simulink model "crossroad_cs_old"  (R2021a)
settings: Solver=ode5  StartTime=0.0  StopTime=50  FixedStep=1/1000  RelTol=1e-3
PreLoadFcn:
  | mbxruntime.callbacks.PreLoadFcn(bdroot);
PostLoadFcn:
  | mbxruntime.callbacks.PostLoadFcn(bdroot);
InitFcn:
  | mbxruntime.callbacks.InitFcn(bdroot);
StartFcn:
  | mbxruntime.callbacks.StartFcn(bdroot);
StopFcn:
  | mbxruntime.callbacks.StopFcn(bdroot);
model workspace: external: MAT-File .\crossroad_cs_hws.mat (data not in the file)
values from neighbouring files (symbols this model uses):
  c_factor = 43.75    [emplanner_init.m]
  cf = -175016    [emplanner_init.m]
  cr = -130634    [emplanner_init.m]
  KD_PID_distance = 0.0    (= 0)    [emplanner_init.m]
  KD_PID_speed = 0    [emplanner_init.m]
  KI_PID_distance = 0.0    (= 0)    [emplanner_init.m]
  KI_PID_speed = 0    [emplanner_init.m]
  KP_PID_distance = 0.5    [emplanner_init.m]
  KP_PID_speed = 1.8    [emplanner_init.m]
  la = 1.265    [emplanner_init.m]
  lb = 2.947-1.265    (= 1.682)    [emplanner_init.m]
  LQR_K1 = k(:,1)'    [emplanner_init.m]
  LQR_K2 = k(:,2)'    [emplanner_init.m]
  LQR_K3 = k(:,3)'    [emplanner_init.m]
  LQR_K4 = k(:,4)'    [emplanner_init.m]
  m = 2020    [emplanner_init.m]
  my_global_path_x = [0.4409 0.940746626271 1.44028225507 1.93950267328 2.43840536558 2.93698884522 3.43525224935 3.93319509352 4.43081712279 4.92811822143 5.42509835808 5.92175755256 ... (6001 elements, 6001x1)]    [my_global_path.mat]    (also in my_global_path_200.mat = [0.4409 0.940746626271 1.44028225507 1.93950267328 2.4384053)
  my_global_path_y = [58.2244 58.2243999975 58.2243999675 58.2243998683 58.224399668 58.2243993499 58.2243989099 58.2243983526 58.2243976886 58.2243969324 58.2243961011 58.2243952132 ... (6001 elements, 6001x1)]    [my_global_path.mat]    (also in my_global_path_200.mat = [58.2244 58.2243999975 58.2243999675 58.2243998683 58.224399)
  rack_displacement = [-39.14 , -37.2 , -35.29 , -33.43 , -31.6 , -29.81 , -28.06 , -26.34 , -24.66 ,      -23.01 , -21.38 , -19.79 , -18.23 , -16.69 , -15.18 , -13.7 , -12.23 , -10.8 , -9.38 , -7.98 ,     -6.61 , -5.25 , -3.91 , -2.59 , -1.29 , 0 , 1.27 , 2.54 , 3.78 , 5.02 , 6.24 , 7.46 , 8.66 ,      9.86 , 11.05 , 12.24 , 13.41 , 14.59 , 15.76 , 16.92 , 18.09 , 19.25 , 20.42 , 21.59 , 22.76 ,      23.93 , 25.11 , 26 ...(+26 chars)    [emplanner_init.m]
  right_wheel_ground = [-70 ,-67.2 , -64.4 , -61.6 , -58.8 , -56 , -53.2 , -50.4 , -47.6 , -44.8 , -42 ,      -39.2 , -36.4 , -33.6 , -30.8 , -28 , -25.2 , -22.4 , -19.6 , -16.8 , -14 , -11.2 , -8.4 , -5.6 ,      -2.8 , 0 , 2.8 , 5.6 , 8.4 , 11.2 , 14 , 16.8 , 19.6 , 22.4 , 25.2 , 28 , 30.8 , 33.6 , 36.4 ,      39.2 , 42 , 44.8 , 47.6 , 50.4 , 53.2 , 56 , 58.8 , 61.6 , 64.4 , 67.2 , 70 ]    [emplanner_init.m]
  vx_break_point = zeros(1,5000)    [emplanner_init.m]
undefined symbols (not defined in the file or in its folder): aubr, DiscIntNeverNeededParam, tablebr, vubr
libraries: PreScanSimulinkLibrary x11, Solver_SF x1
(part 3 of 8)

== system crossroad_cs_old/Audi_A8_Sedan_1/Dynamics_UserSpecified/MuxState ==
  note: mode: Dynamics
  note: mode: Positioning
  note: mode: Dynamics
      | VelVEHICLE
      | wrt VEH
  note: AnglesVEHICLE
      | wrtGLOB
  note: For state mode 'Dynamic' positions
      | are not taken into account, as they
      | are computed by integrating velocity.
      | Click annotation for Help.
  x [m] : Inport  SampleTime=TimeStep
  y [m] : Inport  Port=2  SampleTime=TimeStep
  z [m] : Inport  Port=3  SampleTime=TimeStep
  dx [m/s] : Inport  Port=4  SampleTime=TimeStep
  dy [m/s] : Inport  Port=5  SampleTime=TimeStep
  dz [m/s] : Inport  Port=6  SampleTime=TimeStep
  R [rad] : Inport  Port=7  SampleTime=TimeStep
  P [rad] : Inport  Port=8  SampleTime=TimeStep
  Y [rad] : Inport  Port=9  SampleTime=TimeStep
  Constant : Constant  DisableCoverage=on  Value=positioningmode
  Discrete-Time Integrator : DiscreteIntegrator  SampleTime=TimeStep  ICPrevOutput=DiscIntNeverNeededParam  ICPrevScaledInput=DiscIntNeverNeededParam
  Ground : Ground
  Ground1 : Ground
  Mux1 : Mux  Inputs=[3 3]
  Mux2 : Mux  Inputs=3
  Mux3 : Mux  Inputs=3
  Mux4 : Mux  Inputs=3
  Mux5 : Mux  Inputs=[3 3]
  Mux6 : Mux  Inputs=[6 3]
  Switch : Switch  Threshold=0.5
  Transformation_BODY2GLOBAL : PreScanSimulinkLibrary/Simple_Vehicle_Dynamics/Chassis/MuxDynState/Transformation_BODY2GLOBAL  SystemSampleTime=-1  VariantActivationTime=update diagram  Latency=0  AutoFrameSizeCalculation=off
  mux3 : Mux  Inputs=3
  state : Outport
  wires:
  Constant/1 -> Switch/2
  Mux6/1 -> state/1
  Mux4/1 -> Mux1/1
  Mux5/1 -> Switch/3
  Mux1/1 -> Switch/1
  Switch/1 -> Mux6/1  "PosVeh wrt  GLOB"
  P [rad]/1 -> Mux3/2
  R [rad]/1 -> Mux3/1
  dz [m/s]/1 -> Mux2/3
  dy [m/s]/1 -> Mux2/2
  dx [m/s]/1 -> Mux2/1
  z [m]/1 -> Mux4/3
  y [m]/1 -> Mux4/2
  x [m]/1 -> Mux4/1
  Ground1/1 -> mux3/2  "pitch"
  Y [rad]/1 -> mux3/3, Mux3/3  "yaw"
  Mux3/1 -> Mux6/2
  Transformation_BODY2GLOBAL/1 -> Discrete-Time Integrator/1, Mux5/2  "VelVEH wrt  GLOB"
  mux3/1 -> Transformation_BODY2GLOBAL/2
  Ground/1 -> mux3/1  "roll"
  Mux2/1 -> Mux1/2, Transformation_BODY2GLOBAL/1
  Discrete-Time Integrator/1 -> Mux5/1  "PosVEH wrt  GLOB"

== system crossroad_cs_old/Audi_A8_Sedan_1/Dynamics_UserSpecified/STATE_Audi_A8_Sedan_1 ==
  State : Inport  SampleTime=TimeStep
  Bus Creator : BusCreator  Inputs=15  OutDataTypeStr=Bus: PRESCAN_STATEACTUATORDATA  NonVirtualBus=on
  Constant : Constant  Value=0
  Demux : Demux  Outputs=15
  Mux : Mux  Inputs=3
  Mux1 : Mux  Inputs=3
  Mux2 : Mux  Inputs=3
  iniBODYAngles wrtVEH [rad] : Constant  Value=Roll0  SampleTime=TimeStep
  iniBODYAngles wrtVEH [rad]1 : Constant  Value=Pitch0  SampleTime=TimeStep
  iniVEHAngles wrtGLOB [rad] : Constant  Value=Yaw0  SampleTime=TimeStep
  iniVEHposition wrtGLOB [m] : Constant  Value=x0  SampleTime=TimeStep
  iniVEHposition wrtGLOB [m]1 : Constant  Value=y0  SampleTime=TimeStep
  iniVEHposition wrtGLOB [m]2 : Constant  Value=z0  SampleTime=TimeStep
  state2FullState : PreScanSimulinkLibrary/state2FullState  SystemSampleTime=-1  VariantActivationTime=update diagram  Latency=0  AutoFrameSizeCalculation=off
  StateBus : Outport  OutDataTypeStr=Bus: PRESCAN_STATEACTUATORDATA
  wires:
  Mux2/1 -> state2FullState/4
  iniVEHAngles wrtGLOB [rad]/1 -> Mux2/3
  Mux1/1 -> state2FullState/3
  Constant/1 -> Mux2/1, Mux2/2, Mux1/3
  iniBODYAngles wrtVEH [rad]1/1 -> Mux1/2
  iniBODYAngles wrtVEH [rad]/1 -> Mux1/1
  Mux/1 -> state2FullState/2
  iniVEHposition wrtGLOB [m]2/1 -> Mux/3
  iniVEHposition wrtGLOB [m]/1 -> Mux/1
  iniVEHposition wrtGLOB [m]1/1 -> Mux/2
  Demux/15 -> Bus Creator/15  "AngularVelocityYaw"
  Demux/14 -> Bus Creator/14  "AngularVelocityPitch"
  Demux/13 -> Bus Creator/13  "AngularVelocityRoll"
  Demux/12 -> Bus Creator/12  "OrientationYaw"
  Demux/11 -> Bus Creator/11  "OrientationPitch"
  Demux/10 -> Bus Creator/10  "OrientationRoll"
  Demux/9 -> Bus Creator/9  "AccelerationZ"
  Demux/8 -> Bus Creator/8  "AccelerationY"
  Demux/7 -> Bus Creator/7  "AccelerationX"
  Demux/6 -> Bus Creator/6  "VelocityZ"
  Demux/5 -> Bus Creator/5  "VelocityY"
  Demux/4 -> Bus Creator/4  "VelocityX"
  Demux/3 -> Bus Creator/3  "PositionZ"
  Demux/2 -> Bus Creator/2  "PositionY"
  Demux/1 -> Bus Creator/1  "PositionX"
  state2FullState/1 -> Demux/1
  State/1 -> state2FullState/1
  Bus Creator/1 -> StateBus/1

== system crossroad_cs_old/Audi_A8_Sedan_1/SELF_Demux/compas converter ==
  rotz [rad] : Inport
  cart2compas : Subsystem
  rad2deg : Gain  Gain=180/pi
  heading [deg] : Outport
  wires:
  rad2deg/1 -> cart2compas/1(Angle [deg])
  rotz [rad]/1 -> rad2deg/1
  cart2compas/1(heading [deg]) -> heading [deg]/1

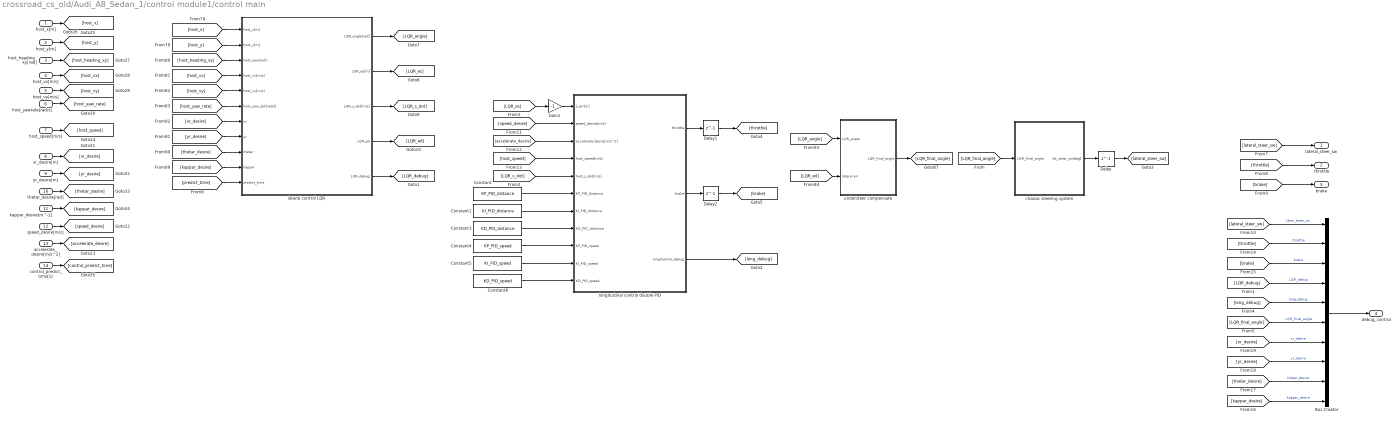
== system crossroad_cs_old/Audi_A8_Sedan_1/control module1/control main ==
  host_x[m] : Inport
  host_y[m] : Inport  Port=2
  host_heading_xy[rad] : Inport  Port=3
  host_vx[m/s] : Inport  Port=4
  host_vy[m/s] : Inport  Port=5
  host_yawrate[rad/s] : Inport  Port=6
  host_speed[m/s] : Inport  Port=7
  xr_desire[m] : Inport  Port=8
  yr_desire[m] : Inport  Port=9
  thetar_desire[rad] : Inport  Port=10
  kappar_desire[m^-1] : Inport  Port=11
  speed_desire[m/s] : Inport  Port=12
  accelerate_desire[m/s^2] : Inport  Port=13
  control_predict_time[s] : Inport  Port=14
  Bus Creator : BusCreator  Inputs=10
  Constant : Constant  Value=KP_PID_distance
  Constant1 : Constant  Value=KI_PID_distance
  Constant3 : Constant  Value=KD_PID_distance
  Constant4 : Constant  Value=KP_PID_speed
  Constant5 : Constant  Value=KI_PID_speed
  Constant6 : Constant  Value=KD_PID_speed
  Delay : Delay  DelayLength=1
  Delay1 : Delay  DelayLength=1
  Delay2 : Delay  DelayLength=1
  Gain2 : Gain  Gain=-1
  chassic steering system : Subsystem
  lateral control LQR : Subsystem
  longitudinal control double PID : Subsystem
  understeer compensate : Subsystem
  lateral_steer_sw : Outport
  throttle : Outport  Port=2
  brake : Outport  Port=3
  debug_control : Outport  Port=4
  wires:
  host_x[m]/1 -> [host_x]
  understeer compensate/1(LQR_final_angle) -> [LQR_final_angle]
  lateral control LQR/1(LQR_angle[rad]) -> [LQR_angle]
  [host_vx] -> lateral control LQR/4(host_vx[m/s])
  thetar_desire[rad]/1 -> [thetar_desire]
  Constant1/1 -> longitudinal control double PID/7(KI_PID_distance)
  [accelerate_desire] -> longitudinal control double PID/3(accelerate desire[m/s^2])
  [host_x] -> lateral control LQR/1(host_x[m])
  [xr_desire] -> lateral control LQR/7(xr)
  accelerate_desire[m/s^2]/1 -> [accelerate_desire]
  [host_y] -> lateral control LQR/2(host_y[m])
  [LQR_s_dot] -> longitudinal control double PID/5(host_s_dot[m/s])
  [yr_desire] -> lateral control LQR/8(yr)
  [LQR_angle] -> understeer compensate/1(LQR_angle)
  xr_desire[m]/1 -> [xr_desire]
  [host_vy] -> lateral control LQR/5(host_vy[m/s])
  lateral control LQR/2(LQR_es[m]) -> [LQR_es]
  host_heading_xy[rad]/1 -> [host_heading_xy]
  [LQR_ed] -> understeer compensate/2(lateral err)
  lateral control LQR/3(LQR_s_dot[m/s]) -> [LQR_s_dot]
  Constant/1 -> longitudinal control double PID/6(KP_PID_distance)
  Constant3/1 -> longitudinal control double PID/8(KD_PID_distance)
  Constant5/1 -> longitudinal control double PID/10(KI_PID_speed)
  Constant4/1 -> longitudinal control double PID/9(KP_PID_speed)
  [host_speed] -> longitudinal control double PID/4(host_speed[m/s])
  [predict_time] -> lateral control LQR/11(predict_time)
  host_vx[m/s]/1 -> [host_vx]
  [speed_desire] -> longitudinal control double PID/2(speed_desire[m/s])
  lateral control LQR/4(LQR_ed) -> [LQR_ed]
  [thetar_desire] -> lateral control LQR/9(thetar)
  [host_heading_xy] -> lateral control LQR/3(host_yaw[rad])
  [kappar_desire] -> lateral control LQR/10(kappar)
  host_yawrate[rad/s]/1 -> [host_yaw_rate]
  kappar_desire[m^-1]/1 -> [kappar_desire]
  yr_desire[m]/1 -> [yr_desire]
  [host_yaw_rate] -> lateral control LQR/6(host_yaw_dot[rad/s])
  host_y[m]/1 -> [host_y]
  host_vy[m/s]/1 -> [host_vy]
  host_speed[m/s]/1 -> [host_speed]
  control_predict_time[s]/1 -> [control_predict_time]
  speed_desire[m/s]/1 -> [speed_desire]
  Constant6/1 -> longitudinal control double PID/11(KD_PID_speed)
  Gain2/1 -> longitudinal control double PID/1(s_err[m])
  [LQR_es] -> Gain2/1
  [LQR_final_angle] -> chassic steering system/1(LQR_final_angle)
  chassic steering system/1(lat_steer_sw[deg]) -> Delay/1
  longitudinal control double PID/1(throttle) -> Delay1/1
  longitudinal control double PID/2(brake) -> Delay2/1
  lateral control LQR/5(LQR_debug) -> [LQR_debug]
  longitudinal control double PID/3(longitudinal_debug) -> [long_debug]
  Delay/1 -> [lateral_steer_sw]
  Delay1/1 -> [throttle]
  Delay2/1 -> [brake]
  [lateral_steer_sw] -> lateral_steer_sw/1
  [throttle] -> throttle/1
  [brake] -> brake/1
  [lateral_steer_sw] -> Bus Creator/1  "later_steer_sw"
  [throttle] -> Bus Creator/2  "throttle"
  [brake] -> Bus Creator/3  "brake"
  [LQR_debug] -> Bus Creator/4  "LQR_debug"
  [long_debug] -> Bus Creator/5  "long_debug"
  [LQR_final_angle] -> Bus Creator/6  "LQR_final_angle"
  Bus Creator/1 -> debug_control/1
  [xr_desire] -> Bus Creator/7  "xr_desire"
  [yr_desire] -> Bus Creator/8  "yr_desire"
  [thetar_desire] -> Bus Creator/9  "thetar_desire"
  [kappar_desire] -> Bus Creator/10  "kappar_desire"

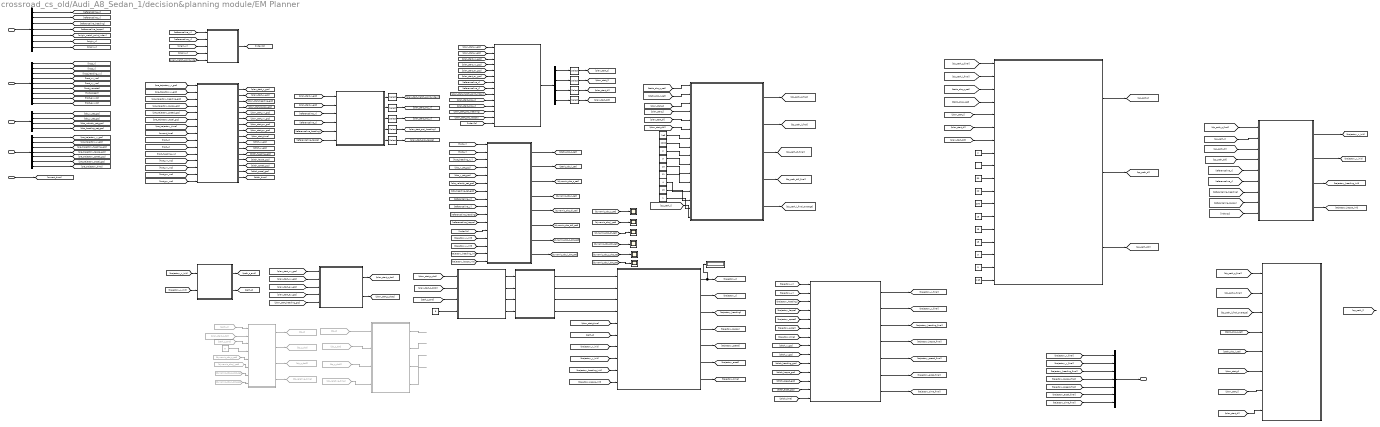
== system crossroad_cs_old/Audi_A8_Sedan_1/decision&planning module/EM Planner ==
  note: ST dynamic programming
  note: output length of curve
  note: Here it should be in global coordinate system
  note: Here it should be in global coordinate system
  referenceline info : Inport
  location info : Inport  Port=2
  perception info : Inport  Port=3
  pre_planning info : Inport  Port=4
  current time : Inport  Port=5
  " " : MATLAB Function  Tag=output length of curve  TreatAsAtomicUnit=on
  Bus Creator : BusCreator  Inputs=7
  Bus Selector : BusSelector  OutputSignals=referenceline_x,referenceline_y,referenceline_heading,referenceline_kappa,origin_match_point_index,origin_x,origin_y
  Bus Selector1 : BusSelector  OutputSignals=host_x,host_y,host_heading_xy,host_vx,host_vy,host_yawrate,host_speed,host_ax,host_ay
  Bus Selector2 : BusSelector  OutputSignals=obs_x_set_gcs,obs_y_set_gcs,obs_velocity_set_gcs,obs_heading_set_gcs
  Bus Selector3 : BusSelector  OutputSignals=trajectory_x_gcs,trajectory_y_gcs,trajectory_heading_gcs,trajectory_kappa_gcs,trajectory_speed_gcs,trajectory_accel_gcs,trajectory_time_gcs
  Bus Selector4 : BusSelector  OutputSignals=s_set,l_set,dl_set,ddl_set
  "Calculate match point index and projection info " : MATLAB Function  TreatAsAtomicUnit=on
  Cartesian2Frenet : Subsystem
  Constant1 : Constant  Commented=on  Value=8
  Constant10 : Constant  Value=1e6
  Constant11 : Constant  Value=2000
  Constant12 : Constant  Value=2
  Constant13 : Constant  Value=25000
  Constant14 : Constant  Value=50
  Constant15 : Constant  Value=20
  Constant16 : Constant  Value=250
  Constant{17..19,28} (4 alike) : Constant  Value=15
  Constant20 : Constant  Value=2
  Constant21 : Constant  Value=3
  Constant22 : Constant  Value=3
  Constant23 : Constant  Value=1.63
  Constant24 : Constant  Value=3
  Constant25 : Constant  Value=10
  Constant26 : Constant  Value=11
  Constant27 : Constant  Value=4
  Constant29 : Constant
  Constant9 : Constant  Value=8
  Display : Display
  Frenet2Cartesian : MATLAB Function  TreatAsAtomicUnit=on
  From123 : From  Commented=on  GotoTag=dp_relative_time
  From134 : From  Commented=on  GotoTag=dynamic_obs_s_dot_set
  From135 : From  Commented=on  GotoTag=dynamic_obs_l_dot_set
  From59 : From  Commented=on  GotoTag=path_s_end
  From60 : From  Commented=on  GotoTag=path_s
  From61 : From  Commented=on  GotoTag=plan_start_s_dot
  From62 : From  Commented=on  GotoTag=dp_s
  From64 : From  Commented=on  GotoTag=dynamic_obs_s_set
  From65 : From  Commented=on  GotoTag=dynamic_obs_l_set
  From66 : From  Commented=on  GotoTag=dp_s_dot
  From67 : From  Commented=on  GotoTag=dp_s_dot2
  Goto92 : Goto  Commented=on  GotoTag=dp_s
  Goto93 : Goto  Commented=on  GotoTag=dp_s_dot
  Goto94 : Goto  Commented=on  GotoTag=dp_s_dot2
  Goto95 : Goto  Commented=on  GotoTag=dp_relative_time
  ST graph : MATLAB Function  Commented=on  TreatAsAtomicUnit=on
  Scope{,1..5} (6 alike) : Scope
  Selector{1..9} (9 alike) : Selector  InputPortWidth=128  IndexOptions=Index vector (dialog)  Indices=1  OutputSizes=1
  calc path length and map between point and s : MATLAB Function  TreatAsAtomicUnit=on
  calc plan start info and stitch trajectory : MATLAB Function  TreatAsAtomicUnit=on
  calc speed planning start condition : MATLAB Function  TreatAsAtomicUnit=on
  increase st point count : MATLAB Function  TreatAsAtomicUnit=on
  increase st point count1 : MATLAB Function  Commented=on  TreatAsAtomicUnit=on
  obs : Subsystem
  path and speed merge : MATLAB Function  TreatAsAtomicUnit=on
  path decision task : Subsystem
  path planning task : Subsystem
  plot : MATLAB Function  TreatAsAtomicUnit=on
  simple speed qp planning : MATLAB Function  TreatAsAtomicUnit=on
  stitch trajectory : MATLAB Function  TreatAsAtomicUnit=on
  EM Planner result : Outport
  wires:
  referenceline info/1 -> Bus Selector/1
  location info/1 -> Bus Selector1/1
  perception info/1 -> Bus Selector2/1
  pre_planning info/1 -> Bus Selector3/1
  current time/1 -> [current_time]
  Bus Selector3/1 -> [pre_trajectory_x_gcs]  "<trajectory_x_gcs>"
  Bus Selector3/2 -> [pre_trajectory_y_gcs]  "<trajectory_y_gcs>"
  Bus Selector3/3 -> [pre_trajectory_heading_gcs]  "<trajectory_heading_gcs>"
  Bus Selector3/4 -> [pre_trajectory_kappa_gcs]  "<trajectory_kappa_gcs>"
  Bus Selector3/5 -> [pre_trajectory_speed_gcs]  "<trajectory_speed_gcs>"
  Bus Selector3/6 -> [pre_trajectory_accel_gcs]  "<trajectory_accel_gcs>"
  Bus Selector3/7 -> [pre_trajectory_time]  "<trajectory_time_gcs>"
  Bus Selector2/1 -> [obs_x_set_gcs]  "<obs_x_set_gcs>"
  Bus Selector2/2 -> [obs_y_set_gcs]  "<obs_y_set_gcs>"
  Bus Selector2/3 -> [obs_velocity_set_gcs]  "<obs_velocity_set_gcs>"
  Bus Selector2/4 -> [obs_heading_set_gcs]  "<obs_heading_set_gcs>"
  Bus Selector1/1 -> [host_x]  "<host_x>"
  Bus Selector1/2 -> [host_y]  "<host_y>"
  Bus Selector1/3 -> [host_heading_xy]  "<host_heading_xy>"
  Bus Selector1/4 -> [host_vx_vcs]  "<host_vx>"
  Bus Selector1/5 -> [host_vy_vcs]  "<host_vy>"
  Bus Selector1/6 -> [host_yawrate]  "<host_yawrate>"
  Bus Selector1/7 -> [host_speed]  "<host_speed>"
  Bus Selector1/8 -> [host_ax_vcs]  "<host_ax>"
  Bus Selector1/9 -> [host_ay_vcs]  "<host_ay>"
  Bus Selector/1 -> [referenceline_x]  "<referenceline_x>"
  Bus Selector/2 -> [referenceline_y]  "<referenceline_y>"
  Bus Selector/3 -> [referenceline_heading]  "<referenceline_heading>"
  Bus Selector/4 -> [referenceline_kappa]  "<referenceline_kappa>"
  [host_ay_vcs] -> calc plan start info and stitch trajectory/15(host_ay)
  [host_ax_vcs] -> calc plan start info and stitch trajectory/14(host_ax)
  [host_vy_vcs] -> calc plan start info and stitch trajectory/13(host_vy)
  [host_vx_vcs] -> calc plan start info and stitch trajectory/12(host_vx)
  [host_heading_xy] -> calc plan start info and stitch trajectory/11(host_heading_xy)
  [host_y] -> calc plan start info and stitch trajectory/10(host_y)
  [host_x] -> calc plan start info and stitch trajectory/9(host_x)
  [current_time] -> calc plan start info and stitch trajectory/8(current_time)
  [pre_trajectory_x_gcs] -> calc plan start info and stitch trajectory/1(pre_trajectory_x)
  [pre_trajectory_y_gcs] -> calc plan start info and stitch trajectory/2(pre_trajectory_y)
  [pre_trajectory_time] -> calc plan start info and stitch trajectory/7(pre_trajectory_time)
  [pre_trajectory_accel_gcs] -> calc plan start info and stitch trajectory/6(pre_trajectory_accel)
  [pre_trajectory_speed_gcs] -> calc plan start info and stitch trajectory/5(pre_trajectory_velocity)
  [pre_trajectory_kappa_gcs] -> calc plan start info and stitch trajectory/4(pre_trajectory_kappa)
  [pre_trajectory_heading_gcs] -> calc plan start info and stitch trajectory/3(pre_trajectory_heading)
  calc plan start info and stitch trajectory/1(plan_start_x) -> [plan_start_x_gcs]
  calc plan start info and stitch trajectory/2(plan_start_y) -> [plan_start_y_gcs]
  calc plan start info and stitch trajectory/3(plan_start_heading) -> [plan_start_heading_gcs]
  calc plan start info and stitch trajectory/4(plan_start_kappa) -> [plan_start_kappa_gcs]
  calc plan start info and stitch trajectory/5(plan_start_vx) -> [plan_start_vx_gcs]
  calc plan start info and stitch trajectory/6(plan_start_vy) -> [plan_start_vy_gcs]
  calc plan start info and stitch trajectory/7(plan_start_ax) -> [plan_start_ax_gcs]
  calc plan start info and stitch trajectory/8(plan_start_ay) -> [plan_start_ay_gcs]
  calc plan start info and stitch trajectory/9(plan_start_time) -> [plan_start_time]
  calc plan start info and stitch trajectory/10(stitch_x) -> [stitch_x_gcs]
  calc plan start info and stitch trajectory/11(stitch_y) -> [stitch_y_gcs]
  calc plan start info and stitch trajectory/12(stitch_heading) -> [stitch_heading_gcs]
  calc plan start info and stitch trajectory/13(stitch_kappa) -> [stitch_kappa_gcs]
  calc plan start info and stitch trajectory/14(stitch_speed) -> [stitch_speed_gcs]
  calc plan start info and stitch trajectory/15(stitch_accel) -> [stitch_accel_gcs]
  calc plan start info and stitch trajectory/16(stitch_time) -> [stitch_time]
  Bus Selector/5 -> [origin_match_point_index]  "<origin_match_point_index>"
  Bus Selector/6 -> [origin_x]  "<origin_x>"
  Bus Selector/7 -> [origin_y]  "<origin_y>"
  [referenceline_x] -> " "/1(path_x)
  [referenceline_y] -> " "/2(path_y)
  [origin_x] -> " "/3(origin_x)
  [origin_y] -> " "/4(origin_y)
  [origin_match_point_index] -> " "/5(origin_match_point_index)
  " "/1(index2s) -> [index2s]
  "Calculate match point index and projection info "/5(proj_kappa_set) -> Selector5/1
  "Calculate match point index and projection info "/3(proj_y_set) -> Selector3/1
  "Calculate match point index and projection info "/1(match_point_index_set) -> Selector1/1
  "Calculate match point index and projection info "/4(proj_heading_set) -> Selector4/1
  "Calculate match point index and projection info "/2(proj_x_set) -> Selector2/1
  [plan_start_x_gcs] -> "Calculate match point index and projection info "/1(x_set)
  [plan_start_y_gcs] -> "Calculate match point index and projection info "/2(y_set)
  [referenceline_x] -> "Calculate match point index and projection info "/3(frenet_path_x)
  [referenceline_y] -> "Calculate match point index and projection info "/4(frenet_path_y)
  [referenceline_heading] -> "Calculate match point index and projection info "/5(frenet_path_heading)
  [referenceline_kappa] -> "Calculate match point index and projection info "/6(frenet_path_kappa)
  Selector1/1 -> [plan_start_match_point_index]
  Selector2/1 -> [plan_start_proj_x]
  Selector3/1 -> [plan_start_proj_y]
  Selector4/1 -> [plan_start_proj_heading]
  Selector5/1 -> [plan_start_proj_kappa]
  [plan_start_y_gcs] -> Cartesian2Frenet/2(y_set)
  [plan_start_x_gcs] -> Cartesian2Frenet/1(x_set)
  [plan_start_vx_gcs] -> Cartesian2Frenet/3(vx_set)
  [plan_start_vy_gcs] -> Cartesian2Frenet/4(vy_set)
  [plan_start_ax_gcs] -> Cartesian2Frenet/5(ax_set)
  [plan_start_ay_gcs] -> Cartesian2Frenet/6(ay_set)
  [referenceline_x] -> Cartesian2Frenet/7(frenet_path_x)
  [referenceline_y] -> Cartesian2Frenet/8(frenet_path_y)
  [plan_start_match_point_index] -> Cartesian2Frenet/9(proj_match_point_index_set)
  [plan_start_proj_x] -> Cartesian2Frenet/10(proj_x_set)
  [plan_start_proj_y] -> Cartesian2Frenet/11(proj_y_set)
  [plan_start_proj_heading] -> Cartesian2Frenet/12(proj_heading_set)
  [plan_start_proj_kappa] -> Cartesian2Frenet/13(proj_kappa_set)
  Cartesian2Frenet/1(Cartesian2FrenetOut) -> Bus Selector4/1
  Bus Selector4/4 -> Selector9/1  "<ddl_set>"
  Bus Selector4/3 -> Selector8/1  "<dl_set>"
  Bus Selector4/2 -> Selector7/1  "<l_set>"
  Bus Selector4/1 -> Selector6/1  "<s_set>"
  Selector6/1 -> [plan_start_s]
  Selector7/1 -> [plan_start_l]
  Selector8/1 -> [plan_start_dl]
  Selector9/1 -> [plan_start_ddl]
  [index2s] -> Cartesian2Frenet/14(index2s)
  [host_x] -> obs/1(host_x)
  [host_y] -> obs/2(host_y)
  [host_heading_xy] -> obs/3(host_heading_xy)
  [obs_x_set_gcs] -> obs/4(obs_x_set_gcs)
  [obs_y_set_gcs] -> obs/5(obs_y_set_gcs)
  [obs_velocity_set_gcs] -> obs/6(obs_velocity_set_gcs)
  [obs_heading_set_gcs] -> obs/7(obs_heading_set_gcs)
  [referenceline_x] -> obs/8(referenceline_x)
  [referenceline_y] -> obs/9(referenceline_y)
  [referenceline_heading] -> obs/10(referenceline_heading)
  [referenceline_kappa] -> obs/11(referenceline_kappa)
  [index2s] -> obs/12(index2s)
  obs/1(static_obs_s_set) -> [static_obs_s_set]
  obs/2(static_obs_l_set) -> [static_obs_l_set]
  path and speed merge/7(trajectory_time) -> [trajectory_time]
  path and speed merge/1(trajectory_x) -> Display/1, [trajectory_x]
  [trajectory_speed] -> stitch trajectory/5(trajectory_speed)
  path and speed merge/4(trajectory_kappa) -> [trajectory_kappa]
  [plan_start_vy_gcs] -> calc speed planning start condition/2(plan_start_vy)
  [stitch_time] -> stitch trajectory/14(stitch_time)
  calc path length and map between point and s/2(path_s) -> [path_s]
  [plan_start_heading_gcs] -> calc speed planning start condition/5(plan_start_heading)
  simple speed qp planning/2(s_dot_init) -> increase st point count/2(s_dot_init)
  Bus Creator/1 -> EM Planner result/1
  simple speed qp planning/1(s_init) -> increase st point count/1(s_init)
  [trajectory_x_final] -> Bus Creator/1  "trajectory_x_gcs"
  stitch trajectory/4(trajectory_kappa_final) -> [trajectory_kappa_final]
  [plan_start_ax_gcs] -> calc speed planning start condition/3(plan_start_ax)
  calc speed planning start condition/1(plan_start_s_dot) -> [plan_start_s_dot]
  [plan_start_ay_gcs] -> calc speed planning start condition/4(plan_start_ay)
  [stitch_speed_gcs] -> stitch trajectory/12(stitch_speed)
  [trajectory_time_final] -> Bus Creator/7  "trajectory_time_gcs"
  Constant9/1 -> simple speed qp planning/4(recommend_T)
  [stitch_x_gcs] -> stitch trajectory/8(stitch_x)
  stitch trajectory/1(trajectory_x_final) -> [trajectory_x_final]
  [trajectory_accel_final] -> Bus Creator/6  "trajectory_accel_gcs"
  [stitch_heading_gcs] -> stitch trajectory/10(stitch_heading)
  [trajectory_speed_final] -> Bus Creator/5  "trajectory_speed_gcs"
  [stitch_y_gcs] -> stitch trajectory/9(stitch_y)
  stitch trajectory/6(trajectory_accel_final) -> [trajectory_accel_final]
  [plan_start_s_dot2] -> simple speed qp planning/2(plan_start_s_dot2)
  [plan_start_vx_gcs] -> calc speed planning start condition/1(plan_start_vx)
  [trajectory_heading_final] -> Bus Creator/3  "trajectory_heading_gcs"
  [trajectory_accel] -> stitch trajectory/6(trajectory_accel)
  [trajectory_kappa] -> stitch trajectory/4(trajectory_kappa)
  stitch trajectory/7(trajectory_time_final) -> [trajectory_time_final]
  [trajectory_x_init] -> path and speed merge/7(trajectory_x_init)
  stitch trajectory/2(trajectory_y_final) -> [trajectory_y_final]
  stitch trajectory/3(trajectory_heading_final) -> [trajectory_heading_final]
  [trajectory_kappa_final] -> Bus Creator/4  "trajectory_kappa_gcs"
  [plan_start_s_dot] -> simple speed qp planning/1(plan_start_s_dot)
  path and speed merge/3(trajectory_heading) -> [trajectory_heading]
  stitch trajectory/5(trajectory_speed_final) -> [trajectory_speed_final]
  [trajectory_y_final] -> Bus Creator/2  "trajectory_y_gcs"
  [trajectory_y] -> stitch trajectory/2(trajectory_y)
  calc path length and map between point and s/1(path_s_end) -> [path_s_end]
  calc speed planning start condition/2(plan_start_s_dot2) -> [plan_start_s_dot2]
  [trajectory_kappa_init] -> path and speed merge/10(trajectory_kappa_init)
  [stitch_accel_gcs] -> stitch trajectory/13(stitch_accel)
  [trajectory_x] -> stitch trajectory/1(trajectory_x)
  [trajectory_y_init] -> calc path length and map between point and s/2(trajectory_y)
  [path_s_end] -> simple speed qp planning/3(s_end)
  path and speed merge/6(trajectory_accel) -> [trajectory_accel]
  [stitch_kappa_gcs] -> stitch trajectory/11(stitch_kappa)
  [path_s] -> path and speed merge/6(path_s)
  path and speed merge/2(trajectory_y) -> [trajectory_y]
  [trajectory_heading_init] -> path and speed merge/9(trajectory_heading_init)
  [plan_start_time] -> path and speed merge/5(current_time)
  path and speed merge/5(trajectory_speed) -> [trajectory_speed]
  simple speed qp planning/4(relative_time_init) -> increase st point count/4(relative_time_init)
  [trajectory_y_init] -> path and speed merge/8(trajectory_y_init)
  [trajectory_time] -> stitch trajectory/7(trajectory_time)
  [trajectory_heading] -> stitch trajectory/3(trajectory_heading)
  [trajectory_x_init] -> calc path length and map between point and s/1(trajectory_x)
  [qp_path_l] -> Frenet2Cartesian/2(l_set)
  [qp_path_dl] -> Frenet2Cartesian/3(dl_set)
  [qp_path_ddl] -> Frenet2Cartesian/4(ddl_set)
  [index2s] -> Frenet2Cartesian/9(index2s)
  [referenceline_x] -> Frenet2Cartesian/5(frenet_path_x)
  [referenceline_y] -> Frenet2Cartesian/6(frenet_path_y)
  [referenceline_heading] -> Frenet2Cartesian/7(frenet_path_heading)
  [referenceline_kappa] -> Frenet2Cartesian/8(frenet_path_kappa)
  Frenet2Cartesian/1(x_set) -> [trajectory_x_init]
  Frenet2Cartesian/2(y_set) -> [trajectory_y_init]
  Frenet2Cartesian/3(heading_set) -> [trajectory_heading_init]
  Frenet2Cartesian/4(kappa_set) -> [trajectory_kappa_init]
  Constant11/1 -> path decision task/8(dp_cost_dl)
  [plan_start_s] -> path decision task/3(plan_start_s)
  path planning task/3(qp_path_ddl) -> [qp_path_ddl]
  Constant24/1 -> path decision task/10(dp_cost_dddl)
  Constant27/1 -> path decision task/13(dp_col)
  Constant15/1 -> path planning task/11(qp_cost_dddl)
  Constant21/1 -> path planning task/16(host_d1)
  Constant16/1 -> path planning task/12(qp_cost_centre)
  Constant26/1 -> path decision task/12(dp_row)
  Constant12/1 -> path planning task/8(qp_cost_l)
  Constant10/1 -> path decision task/7(dp_cost_collision)
  [dp_path_s_final] -> path planning task/1(dp_path_s_final)
  Constant25/1 -> path decision task/11(dp_cost_ref)
  Constant13/1 -> path planning task/9(qp_cost_dl)
  [dp_path_l_final] -> path planning task/2(dp_path_l_final)
  Constant18/1 -> path planning task/14(qp_cost_end_dl)
  Constant28/1 -> path decision task/14(dp_sample_s)
  Constant19/1 -> path planning task/15(qp_cost_end_ddl)
  [plan_start_ddl] -> path planning task/7(plan_start_ddl)
  Constant22/1 -> path planning task/17(host_d2)
  Constant14/1 -> path planning task/10(qp_cost_ddl)
  Constant17/1 -> path planning task/13(qp_cost_endl)
  [plan_start_dl] -> path planning task/6(plan_start_dl)
  path planning task/2(qp_path_dl) -> [qp_path_dl]
  path planning task/1(qp_path_l) -> [qp_path_l]
  [plan_start_l] -> path planning task/5(plan_start_l)
  [static_obs_s_set] -> path planning task/3(static_obs_s_set)
  [plan_start_l] -> path decision task/4(plan_start_l)
  [static_obs_l_set] -> path planning task/4(static_obs_l_set)
  Constant20/1 -> path decision task/9(dp_cost_ddl)
  [plan_start_ddl] -> path decision task/6(plan_start_ddl)
  path decision task/3(dp_path_dl_final) -> [dp_path_dl_final]
  [static_obs_l_set] -> path decision task/2(static_obs_l_set)
  Constant29/1 -> path decision task/15(dp_sample_l)
  path decision task/4(dp_path_ddl_final) -> [dp_path_ddl_final]
  Constant23/1 -> path planning task/18(host_w)
  [plan_start_dl] -> path decision task/5(plan_start_dl)
  path decision task/1(dp_path_s_final) -> [dp_path_s_final]
  [static_obs_s_set] -> path decision task/1(static_obs_s_set)
  path decision task/2(dp_path_l_final) -> [dp_path_l_final]
  [dp_path_s_final] -> Frenet2Cartesian/1(s_set)
  [static_obs_l_set] -> plot/5(obs_l_set)
  [dp_path_l_final] -> plot/2(dp_l)
  [static_obs_s_set] -> plot/4(obs_s_set)
  [plan_start_s] -> plot/6(start_s)
  [dp_path_s_final] -> plot/1(dp_s)
  [plan_start_dl] -> plot/8(start_dl)
  [plan_start_l] -> plot/7(start_l)
  obs/3(dynamic_obs_s_set) -> [dynamic_obs_s_set]
  obs/4(dynamic_obs_l_set) -> [dynamic_obs_l_set]
  obs/5(dynamic_obs_dl_set) -> [dynamic_obs_dl_set]
  [qp_path_l] -> path decision task/16(qp_path_l_in_last_cycle)
  From60/1 -> ST graph/1(path_s)
  Constant1/1 -> ST graph/4(recommended_T)
  [trajectory_y_init] -> obs/14(trajectory_y)
  [trajectory_x_init] -> obs/13(trajectory_x)
  obs/6(dynamic_obs_ddl_set) -> [dynamic_obs_ddl_set]
  obs/7(dynamic_obs_s_dot_set) -> [dynamic_obs_s_dot_set]
  obs/8(dynamic_obs_l_dot_set) -> [dynamic_obs_l_dot_set]
  path decision task/5(dp_path_l_final_average) -> [dp_path_l_final_average]
  [dp_path_l_final_average] -> plot/3(qp_l)
  From59/1 -> ST graph/3(path_s_end)
  From64/1 -> ST graph/5(dynamic_obs_s_set)
  From65/1 -> ST graph/6(dynamic_obs_l_set)
  From134/1 -> ST graph/7(dynamic_obs_s_dot_set)
  From135/1 -> ST graph/8(dynamic_obs_l_dot_set)
  [qp_path_l] -> ?
  [dynamic_obs_s_set] -> Scope/1
  [dynamic_obs_l_set] -> Scope1/1
  [dynamic_obs_dl_set] -> Scope2/1
  [dynamic_obs_ddl_set] -> Scope3/1
  [dynamic_obs_s_dot_set] -> Scope4/1
  [dynamic_obs_l_dot_set] -> Scope5/1
  [trajectory_heading_init] -> obs/15(trajectory_heading)
  [trajectory_kappa_init] -> obs/16(trajectory_kappa)
  From61/1 -> ST graph/2(plan_start_s_dot)
  ST graph/1(dp_s) -> Goto92/1
  ST graph/2(dp_s_dot) -> Goto93/1
  ST graph/3(dp_s_dot2) -> Goto94/1
  ST graph/4(dp_relative_time) -> Goto95/1
  From62/1 -> increase st point count1/1(s_init)
  From66/1 -> increase st point count1/2(s_dot_init)
  From67/1 -> increase st point count1/3(s_dot2_init)
  From123/1 -> increase st point count1/4(relative_time_init)
  increase st point count/2(s_dot) -> path and speed merge/2(s_dot)
  simple speed qp planning/3(s_dot2_init) -> increase st point count/3(s_dot2_init)
  increase st point count1/1(s) -> ?
  increase st point count1/2(s_dot) -> ?
  increase st point count1/3(s_dot2) -> ?
  increase st point count1/4(relative_time) -> ?
  increase st point count/1(s) -> path and speed merge/1(s)
  increase st point count/3(s_dot2) -> path and speed merge/3(s_dot2)
  increase st point count/4(relative_time) -> path and speed merge/4(relative_time)

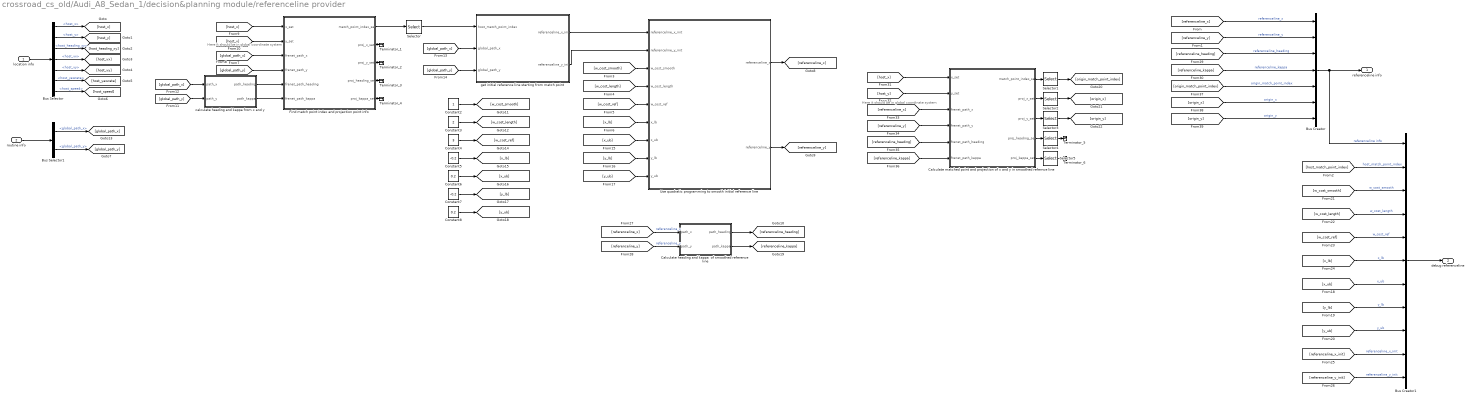
== system crossroad_cs_old/Audi_A8_Sedan_1/decision&planning module/referenceline provider ==
  note: Here it should be in global coordinate system
  note: Here it should be in global coordinate system
  location info : Inport
  routine info : Inport  Port=2
  Bus Creator : BusCreator  Inputs=7
  Bus Creator1 : BusCreator  Inputs=11
  Bus Selector : BusSelector  OutputSignals=host_x,host_y,host_heading_xy,host_vx,host_vy,host_yawrate,host_speed
  Bus Selector1 : BusSelector  OutputSignals=global_path_x,global_path_y
  Calculate heading and kappa  of smoothed reference line : MATLAB Function  TreatAsAtomicUnit=on
  Calculate matched point and projection of x and y in smoothed refernce line : MATLAB Function  TreatAsAtomicUnit=on
  Constant2 : Constant
  Constant3 : Constant  Value=2
  Constant4 : Constant  Value=3
  Constant5 : Constant  Value=-0.2
  Constant6 : Constant  Value=0.2
  Constant7 : Constant  Value=-0.2
  Constant8 : Constant  Value=0.2
  Find match point index and projection point info : MATLAB Function  TreatAsAtomicUnit=on
  Selector{,1..5} (6 alike) : Selector  InputPortWidth=128  IndexOptions=Index vector (dialog)  Indices=1  OutputSizes=1
  Terminator_{1..6} (6 alike) : Terminator
  Use quadratic programming to smooth initial reference line : MATLAB Function  TreatAsAtomicUnit=on
  calculate heading and kappa from x and y : MATLAB Function  TreatAsAtomicUnit=on
  get initial reference line starting from match point : MATLAB Function  TreatAsAtomicUnit=on
  referenceline info : Outport
  debug referenceline : Outport  Port=2
  wires:
  [global_path_x] -> get initial reference line starting from match point/2(global_path_x)
  [host_x] -> Find match point index and projection point info/1(x_set)
  calculate heading and kappa from x and y/2(path_kappa) -> Find match point index and projection point info/6(frenet_path_kappa)
  calculate heading and kappa from x and y/1(path_heading) -> Find match point index and projection point info/5(frenet_path_heading)
  [global_path_y] -> Find match point index and projection point info/4(frenet_path_y)
  [global_path_x] -> Find match point index and projection point info/3(frenet_path_x)
  [host_y] -> Find match point index and projection point info/2(y_set)
  [global_path_y] -> calculate heading and kappa from x and y/2(path_y)
  [global_path_x] -> calculate heading and kappa from x and y/1(path_x)
  Selector/1 -> get initial reference line starting from match point/1(host_match_point_index)
  Find match point index and projection point info/1(match_point_index_set) -> Selector/1
  [global_path_y] -> get initial reference line starting from match point/3(global_path_y)
  get initial reference line starting from match point/1(referenceline_x_init) -> Use quadratic programming to smooth initial reference line/1(referenceline_x_init)
  Bus Selector/5 -> [host_vy]  "<host_vy>"
  Bus Selector/1 -> [host_x]  "<host_x>"
  Bus Selector/2 -> [host_y]  "<host_y>"
  Bus Selector/3 -> [host_heading_xy]  "<host_heading_xy>"
  Bus Selector/4 -> [host_vx]  "<host_vx>"
  Bus Selector/7 -> [host_speed]  "<host_speed>"
  Bus Selector/6 -> [host_yawrate]  "<host_yawrate>"
  location info/1 -> Bus Selector/1
  Bus Selector1/2 -> [global_path_y]  "<global_path_y>"
  Bus Selector1/1 -> [global_path_x]  "<global_path_x>"
  routine info/1 -> Bus Selector1/1
  Use quadratic programming to smooth initial reference line/1(referenceline_x) -> [referenceline_x]
  Use quadratic programming to smooth initial reference line/2(referenceline_y) -> [referenceline_y]
  [referenceline_x] -> Bus Creator/1  "referenceline_x"
  [referenceline_y] -> Bus Creator/2  "referenceline_y"
  Bus Creator1/1 -> debug referenceline/1
  Bus Creator/1 -> Bus Creator1/1, referenceline info/1  "referenceline info"
  Constant2/1 -> [w_cost_smooth]
  Constant3/1 -> [w_cost_length]
  Constant8/1 -> [y_ub]
  Constant7/1 -> [y_lb]
  Constant6/1 -> [x_ub]
  Constant5/1 -> [x_lb]
  Constant4/1 -> [w_cost_ref]
  [w_cost_smooth] -> Use quadratic programming to smooth initial reference line/3(w_cost_smooth)
  [w_cost_length] -> Use quadratic programming to smooth initial reference line/4(w_cost_length)
  [w_cost_ref] -> Use quadratic programming to smooth initial reference line/5(w_cost_ref)
  [x_lb] -> Use quadratic programming to smooth initial reference line/6(x_lb)
  [x_ub] -> Use quadratic programming to smooth initial reference line/7(x_ub)
  [y_lb] -> Use quadratic programming to smooth initial reference line/8(y_lb)
  [y_ub] -> Use quadratic programming to smooth initial reference line/9(y_ub)
  get initial reference line starting from match point/2(referenceline_y_init) -> Use quadratic programming to smooth initial reference line/2(referenceline_y_init)
  [w_cost_ref] -> Bus Creator1/5  "w_cost_ref"
  [x_lb] -> Bus Creator1/6  "x_lb"
  [w_cost_length] -> Bus Creator1/4  "w_cost_length"
  [x_ub] -> Bus Creator1/7  "x_ub"
  [w_cost_smooth] -> Bus Creator1/3  "w_cost_smooth"
  [y_lb] -> Bus Creator1/8  "y_lb"
  [host_match_point_index] -> Bus Creator1/2  "host_match_point_index"
  [y_ub] -> Bus Creator1/9  "y_ub"
  [referenceline_x_init] -> Bus Creator1/10  "referenceline_x_init"
  [referenceline_y_init] -> Bus Creator1/11  "referenceline_y_init"
  [referenceline_x] -> Calculate heading and kappa  of smoothed reference line/1(path_x)  "referenceline_x"
  [referenceline_y] -> Calculate heading and kappa  of smoothed reference line/2(path_y)  "referenceline_y"
  Calculate heading and kappa  of smoothed reference line/1(path_heading) -> [referenceline_heading]
  Calculate heading and kappa  of smoothed reference line/2(path_kappa) -> [referenceline_kappa]
  [referenceline_kappa] -> Bus Creator/4  "referenceline_kappa"
  [referenceline_heading] -> Bus Creator/3  "referenceline_heading"
  [host_x] -> Calculate matched point and projection of x and y in smoothed refernce line/1(x_set)
  [host_y] -> Calculate matched point and projection of x and y in smoothed refernce line/2(y_set)
  [referenceline_x] -> Calculate matched point and projection of x and y in smoothed refernce line/3(frenet_path_x)
  [referenceline_y] -> Calculate matched point and projection of x and y in smoothed refernce line/4(frenet_path_y)
  [referenceline_heading] -> Calculate matched point and projection of x and y in smoothed refernce line/5(frenet_path_heading)
  [referenceline_kappa] -> Calculate matched point and projection of x and y in smoothed refernce line/6(frenet_path_kappa)
  Calculate matched point and projection of x and y in smoothed refernce line/1(match_point_index_set) -> Selector1/1
  Calculate matched point and projection of x and y in smoothed refernce line/2(proj_x_set) -> Selector2/1
  Calculate matched point and projection of x and y in smoothed refernce line/3(proj_y_set) -> Selector3/1
  Calculate matched point and projection of x and y in smoothed refernce line/4(proj_heading_set) -> Selector4/1
  Calculate matched point and projection of x and y in smoothed refernce line/5(proj_kappa_set) -> Selector5/1
  Selector1/1 -> [origin_match_point_index]
  Selector2/1 -> [origin_x]
  Selector3/1 -> [origin_y]
  [origin_match_point_index] -> Bus Creator/5  "origin_match_point_index"
  [origin_x] -> Bus Creator/6  "origin_x"
  [origin_y] -> Bus Creator/7  "origin_y"
  Find match point index and projection point info/2(proj_x_set) -> Terminator_1/1
  Find match point index and projection point info/3(proj_y_set) -> Terminator_2/1
  Find match point index and projection point info/4(proj_heading_set) -> Terminator_3/1
  Find match point index and projection point info/5(proj_kappa_set) -> Terminator_4/1
  Selector4/1 -> Terminator_5/1
  Selector5/1 -> Terminator_6/1

== system crossroad_cs_old/Box_1/Dynamics_Empty/MuxState ==
  note: mode: Dynamics
  note: mode: Positioning
  note: mode: Dynamics
      | VelVEHICLE
      | wrt VEH
  note: AnglesVEHICLE
      | wrtGLOB
  note: For state mode 'Dynamic' positions
      | are not taken into account, as they
      | are computed by integrating velocity.
      | Click annotation for Help.
  x [m] : Inport  SampleTime=TimeStep
  y [m] : Inport  Port=2  SampleTime=TimeStep
  z [m] : Inport  Port=3  SampleTime=TimeStep
  dx [m/s] : Inport  Port=4  SampleTime=TimeStep
  dy [m/s] : Inport  Port=5  SampleTime=TimeStep
  dz [m/s] : Inport  Port=6  SampleTime=TimeStep
  R [rad] : Inport  Port=7  SampleTime=TimeStep
  P [rad] : Inport  Port=8  SampleTime=TimeStep
  Y [rad] : Inport  Port=9  SampleTime=TimeStep
  Constant : Constant  DisableCoverage=on  Value=positioningmode
  Discrete-Time Integrator : DiscreteIntegrator  SampleTime=TimeStep  ICPrevOutput=DiscIntNeverNeededParam  ICPrevScaledInput=DiscIntNeverNeededParam
  Ground : Ground
  Ground1 : Ground
  Mux1 : Mux  Inputs=[3 3]
  Mux2 : Mux  Inputs=3
  Mux3 : Mux  Inputs=3
  Mux4 : Mux  Inputs=3
  Mux5 : Mux  Inputs=[3 3]
  Mux6 : Mux  Inputs=[6 3]
  Switch : Switch  Threshold=0.5
  Transformation_BODY2GLOBAL : PreScanSimulinkLibrary/Simple_Vehicle_Dynamics/Chassis/MuxDynState/Transformation_BODY2GLOBAL  SystemSampleTime=-1  VariantActivationTime=update diagram  Latency=0  AutoFrameSizeCalculation=off
  mux3 : Mux  Inputs=3
  state : Outport
  wires:
  Constant/1 -> Switch/2
  Mux6/1 -> state/1
  Mux4/1 -> Mux1/1
  Mux5/1 -> Switch/3
  Mux1/1 -> Switch/1
  Switch/1 -> Mux6/1  "PosVeh wrt  GLOB"
  P [rad]/1 -> Mux3/2
  R [rad]/1 -> Mux3/1
  dz [m/s]/1 -> Mux2/3
  dy [m/s]/1 -> Mux2/2
  dx [m/s]/1 -> Mux2/1
  z [m]/1 -> Mux4/3
  y [m]/1 -> Mux4/2
  x [m]/1 -> Mux4/1
  Ground1/1 -> mux3/2  "pitch"
  Y [rad]/1 -> mux3/3, Mux3/3  "yaw"
  Mux3/1 -> Mux6/2
  Transformation_BODY2GLOBAL/1 -> Discrete-Time Integrator/1, Mux5/2  "VelVEH wrt  GLOB"
  mux3/1 -> Transformation_BODY2GLOBAL/2
  Ground/1 -> mux3/1  "roll"
  Mux2/1 -> Mux1/2, Transformation_BODY2GLOBAL/1
  Discrete-Time Integrator/1 -> Mux5/1  "PosVEH wrt  GLOB"

== system crossroad_cs_old/Box_1/Dynamics_Empty/STATE_Box_1 ==
  State : Inport  SampleTime=TimeStep
  Bus Creator : BusCreator  Inputs=15  OutDataTypeStr=Bus: PRESCAN_STATEACTUATORDATA  NonVirtualBus=on
  Constant : Constant  Value=0
  Demux : Demux  Outputs=15
  Mux : Mux  Inputs=3
  Mux1 : Mux  Inputs=3
  Mux2 : Mux  Inputs=3
  iniBODYAngles wrtVEH [rad] : Constant  Value=Roll0  SampleTime=TimeStep
  iniBODYAngles wrtVEH [rad]1 : Constant  Value=Pitch0  SampleTime=TimeStep
  iniVEHAngles wrtGLOB [rad] : Constant  Value=Yaw0  SampleTime=TimeStep
  iniVEHposition wrtGLOB [m] : Constant  Value=x0  SampleTime=TimeStep
  iniVEHposition wrtGLOB [m]1 : Constant  Value=y0  SampleTime=TimeStep
  iniVEHposition wrtGLOB [m]2 : Constant  Value=z0  SampleTime=TimeStep
  state2FullState : PreScanSimulinkLibrary/state2FullState  SystemSampleTime=-1  VariantActivationTime=update diagram  Latency=0  AutoFrameSizeCalculation=off
  StateBus : Outport  OutDataTypeStr=Bus: PRESCAN_STATEACTUATORDATA
  wires:
  Mux2/1 -> state2FullState/4
  iniVEHAngles wrtGLOB [rad]/1 -> Mux2/3
  Mux1/1 -> state2FullState/3
  Constant/1 -> Mux2/1, Mux2/2, Mux1/3
  iniBODYAngles wrtVEH [rad]1/1 -> Mux1/2
  iniBODYAngles wrtVEH [rad]/1 -> Mux1/1
  Mux/1 -> state2FullState/2
  iniVEHposition wrtGLOB [m]2/1 -> Mux/3
  iniVEHposition wrtGLOB [m]/1 -> Mux/1
  iniVEHposition wrtGLOB [m]1/1 -> Mux/2
  Demux/15 -> Bus Creator/15  "AngularVelocityYaw"
  Demux/14 -> Bus Creator/14  "AngularVelocityPitch"
  Demux/13 -> Bus Creator/13  "AngularVelocityRoll"
  Demux/12 -> Bus Creator/12  "OrientationYaw"
  Demux/11 -> Bus Creator/11  "OrientationPitch"
  Demux/10 -> Bus Creator/10  "OrientationRoll"
  Demux/9 -> Bus Creator/9  "AccelerationZ"
  Demux/8 -> Bus Creator/8  "AccelerationY"
  Demux/7 -> Bus Creator/7  "AccelerationX"
  Demux/6 -> Bus Creator/6  "VelocityZ"
  Demux/5 -> Bus Creator/5  "VelocityY"
  Demux/4 -> Bus Creator/4  "VelocityX"
  Demux/3 -> Bus Creator/3  "PositionZ"
  Demux/2 -> Bus Creator/2  "PositionY"
  Demux/1 -> Bus Creator/1  "PositionX"
  state2FullState/1 -> Demux/1
  State/1 -> state2FullState/1
  Bus Creator/1 -> StateBus/1

== system crossroad_cs_old/Box_1/SELF_Demux/compas converter ==
  rotz [rad] : Inport
  cart2compas : Subsystem
  rad2deg : Gain  Gain=180/pi
  heading [deg] : Outport
  wires:
  rad2deg/1 -> cart2compas/1(Angle [deg])
  rotz [rad]/1 -> rad2deg/1
  cart2compas/1(heading [deg]) -> heading [deg]/1

== system crossroad_cs_old/Box_2/Dynamics_Empty/MuxState ==
  note: mode: Dynamics
  note: mode: Positioning
  note: mode: Dynamics
      | VelVEHICLE
      | wrt VEH
  note: AnglesVEHICLE
      | wrtGLOB
  note: For state mode 'Dynamic' positions
      | are not taken into account, as they
      | are computed by integrating velocity.
      | Click annotation for Help.
  x [m] : Inport  SampleTime=TimeStep
  y [m] : Inport  Port=2  SampleTime=TimeStep
  z [m] : Inport  Port=3  SampleTime=TimeStep
  dx [m/s] : Inport  Port=4  SampleTime=TimeStep
  dy [m/s] : Inport  Port=5  SampleTime=TimeStep
  dz [m/s] : Inport  Port=6  SampleTime=TimeStep
  R [rad] : Inport  Port=7  SampleTime=TimeStep
  P [rad] : Inport  Port=8  SampleTime=TimeStep
  Y [rad] : Inport  Port=9  SampleTime=TimeStep
  Constant : Constant  DisableCoverage=on  Value=positioningmode
  Discrete-Time Integrator : DiscreteIntegrator  SampleTime=TimeStep  ICPrevOutput=DiscIntNeverNeededParam  ICPrevScaledInput=DiscIntNeverNeededParam
  Ground : Ground
  Ground1 : Ground
  Mux1 : Mux  Inputs=[3 3]
  Mux2 : Mux  Inputs=3
  Mux3 : Mux  Inputs=3
  Mux4 : Mux  Inputs=3
  Mux5 : Mux  Inputs=[3 3]
  Mux6 : Mux  Inputs=[6 3]
  Switch : Switch  Threshold=0.5
  Transformation_BODY2GLOBAL : PreScanSimulinkLibrary/Simple_Vehicle_Dynamics/Chassis/MuxDynState/Transformation_BODY2GLOBAL  SystemSampleTime=-1  VariantActivationTime=update diagram  Latency=0  AutoFrameSizeCalculation=off
  mux3 : Mux  Inputs=3
  state : Outport
  wires:
  Constant/1 -> Switch/2
  Mux6/1 -> state/1
  Mux4/1 -> Mux1/1
  Mux5/1 -> Switch/3
  Mux1/1 -> Switch/1
  Switch/1 -> Mux6/1  "PosVeh wrt  GLOB"
  P [rad]/1 -> Mux3/2
  R [rad]/1 -> Mux3/1
  dz [m/s]/1 -> Mux2/3
  dy [m/s]/1 -> Mux2/2
  dx [m/s]/1 -> Mux2/1
  z [m]/1 -> Mux4/3
  y [m]/1 -> Mux4/2
  x [m]/1 -> Mux4/1
  Ground1/1 -> mux3/2  "pitch"
  Y [rad]/1 -> mux3/3, Mux3/3  "yaw"
  Mux3/1 -> Mux6/2
  Transformation_BODY2GLOBAL/1 -> Discrete-Time Integrator/1, Mux5/2  "VelVEH wrt  GLOB"
  mux3/1 -> Transformation_BODY2GLOBAL/2
  Ground/1 -> mux3/1  "roll"
  Mux2/1 -> Mux1/2, Transformation_BODY2GLOBAL/1
  Discrete-Time Integrator/1 -> Mux5/1  "PosVEH wrt  GLOB"

== system crossroad_cs_old/Box_2/Dynamics_Empty/STATE_Box_2 ==
  State : Inport  SampleTime=TimeStep
  Bus Creator : BusCreator  Inputs=15  OutDataTypeStr=Bus: PRESCAN_STATEACTUATORDATA  NonVirtualBus=on
  Constant : Constant  Value=0
  Demux : Demux  Outputs=15
  Mux : Mux  Inputs=3
  Mux1 : Mux  Inputs=3
  Mux2 : Mux  Inputs=3
  iniBODYAngles wrtVEH [rad] : Constant  Value=Roll0  SampleTime=TimeStep
  iniBODYAngles wrtVEH [rad]1 : Constant  Value=Pitch0  SampleTime=TimeStep
  iniVEHAngles wrtGLOB [rad] : Constant  Value=Yaw0  SampleTime=TimeStep
  iniVEHposition wrtGLOB [m] : Constant  Value=x0  SampleTime=TimeStep
  iniVEHposition wrtGLOB [m]1 : Constant  Value=y0  SampleTime=TimeStep
  iniVEHposition wrtGLOB [m]2 : Constant  Value=z0  SampleTime=TimeStep
  state2FullState : PreScanSimulinkLibrary/state2FullState  SystemSampleTime=-1  VariantActivationTime=update diagram  Latency=0  AutoFrameSizeCalculation=off
  StateBus : Outport  OutDataTypeStr=Bus: PRESCAN_STATEACTUATORDATA
  wires:
  Mux2/1 -> state2FullState/4
  iniVEHAngles wrtGLOB [rad]/1 -> Mux2/3
  Mux1/1 -> state2FullState/3
  Constant/1 -> Mux2/1, Mux2/2, Mux1/3
  iniBODYAngles wrtVEH [rad]1/1 -> Mux1/2
  iniBODYAngles wrtVEH [rad]/1 -> Mux1/1
  Mux/1 -> state2FullState/2
  iniVEHposition wrtGLOB [m]2/1 -> Mux/3
  iniVEHposition wrtGLOB [m]/1 -> Mux/1
  iniVEHposition wrtGLOB [m]1/1 -> Mux/2
  Demux/15 -> Bus Creator/15  "AngularVelocityYaw"
  Demux/14 -> Bus Creator/14  "AngularVelocityPitch"
  Demux/13 -> Bus Creator/13  "AngularVelocityRoll"
  Demux/12 -> Bus Creator/12  "OrientationYaw"
  Demux/11 -> Bus Creator/11  "OrientationPitch"
  Demux/10 -> Bus Creator/10  "OrientationRoll"
  Demux/9 -> Bus Creator/9  "AccelerationZ"
  Demux/8 -> Bus Creator/8  "AccelerationY"
  Demux/7 -> Bus Creator/7  "AccelerationX"
  Demux/6 -> Bus Creator/6  "VelocityZ"
  Demux/5 -> Bus Creator/5  "VelocityY"
  Demux/4 -> Bus Creator/4  "VelocityX"
  Demux/3 -> Bus Creator/3  "PositionZ"
  Demux/2 -> Bus Creator/2  "PositionY"
  Demux/1 -> Bus Creator/1  "PositionX"
  state2FullState/1 -> Demux/1
  State/1 -> state2FullState/1
  Bus Creator/1 -> StateBus/1

== system crossroad_cs_old/Box_2/SELF_Demux/compas converter ==
  rotz [rad] : Inport
  cart2compas : Subsystem
  rad2deg : Gain  Gain=180/pi
  heading [deg] : Outport
  wires:
  rad2deg/1 -> cart2compas/1(Angle [deg])
  rotz [rad]/1 -> rad2deg/1
  cart2compas/1(heading [deg]) -> heading [deg]/1
